simulink model "sf_fxptprecision"  (Simulink 7.6)
settings: Solver=FixedStepDiscrete  StartTime=0.0  StopTime=1  FixedStep=1  RelTol=1e-3
settings Model: Creator=The MathWorks Inc.  CovMetricSettings=dcmtr  ExtModeAutoUpdateStatusClock=off
settings OptimizationCC: InlineInvariantSignals=on  InitFltsAndDblsToZero=on  EfficientMapNaN2IntZero=off
settings DebuggingCC: SaveWithParameterizedLinksMsg=none  SignalResolutionControl=TryResolveAllWithWarning  SolverPrmCheckMsg=none  MultiTaskDSMMsg=warning  MultiTaskCondExecSysMsg=none  StrictBusMsg=None
settings HardwareCC: TargetUnknown=on
settings SFSimCC: SimParseCustomCode=off
settings RTWCC: IncludeERTFirstTime=on
settings GRTTargetCC: TargetFcnLib=ansi_tfl_tmw.mat

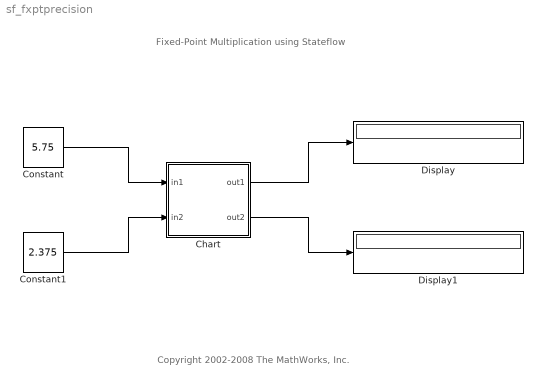
== system sf_fxptprecision ==
  note: Fixed-Point Multiplication using Stateflow
  note: Copyright 2002-2008 The MathWorks, Inc.
  Chart : Stateflow chart  TreatAsAtomicUnit=on
  Constant : Constant  Value=5.75  OutDataTypeStr=fixdt(0,8,2)
  Constant1 : Constant  Value=2.375  OutDataTypeStr=fixdt(0,8,3)
  Display : Display
  Display1 : Display
  wires:
  Constant/1 -> Chart/1(in1)
  Constant1/1 -> Chart/2(in2)
  Chart/1(out1) -> Display/1
  Chart/2(out2) -> Display1/1

== stateflow chart Chart ==
  (default) -> (junction 3) : {out1=in1*in2;}
  (junction 3) -> (junction 4) : {out2=in1*in2;}
  data: in1 input fixdt(0,8,2); in2 input fixdt(0,8,3); out1 output fixdt(0,8,2); out2 output fixdt(0,8,4)
